simulink model "zad4_model"  (R2017a)
settings: Solver=VariableStepAuto  StartTime=0.0  StopTime=2  RelTol=1e-3
values from neighbouring files (symbols this model uses):
  a1 = Ap(1,1)    [zad4.m]
  a2 = Ap(2,1)    [zad4.m]
  a3 = Ap(3,1)    [zad4.m]
  b1 = Bp(1)    [zad4.m]
  b2 = Bp(2)    [zad4.m]
  b3 = Bp(3)    [zad4.m]
  K = acker(A2, B2, [z z z])    [zad3a.m]    (also in zad3b.m = acker(A2, B2, [z1 z2 z2]); zad3max.m; zad4.m = acker(Ap, Bp, [0.6 0.4 0.4]))
  l1 = L(1)    [zad4.m]
  l2 = L(2)    [zad4.m]
  Tp = 0.1    [zad3a.m]    (also in zad3b.m; zad3max.m; zad4.m)
settings Model: Creator=Rajtek  LastModifiedBy=Rajtek

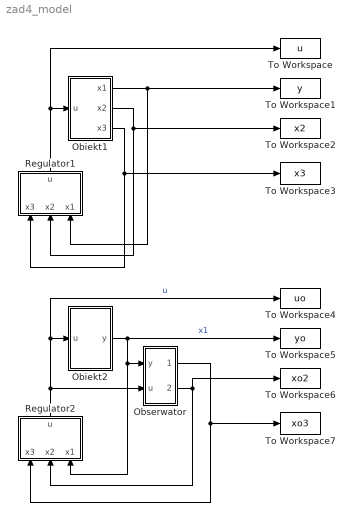
== system zad4_model ==
  Obiekt1 : Subsystem
  Obiekt2 : Subsystem
  Obserwator : Subsystem
  Regulator1 : Subsystem
  Regulator2 : Subsystem
  To Workspace : ToWorkspace  VariableName=u  SaveFormat=Timeseries  SampleTime=-1
  To Workspace1 : ToWorkspace  VariableName=y  SaveFormat=Timeseries  SampleTime=-1
  To Workspace2 : ToWorkspace  VariableName=x2  SaveFormat=Timeseries  SampleTime=-1
  To Workspace3 : ToWorkspace  VariableName=x3  SaveFormat=Timeseries  SampleTime=-1
  To Workspace4 : ToWorkspace  VariableName=uo  SaveFormat=Timeseries  SampleTime=-1
  To Workspace5 : ToWorkspace  VariableName=yo  SaveFormat=Timeseries  SampleTime=-1
  To Workspace6 : ToWorkspace  VariableName=xo2  SaveFormat=Timeseries  SampleTime=-1
  To Workspace7 : ToWorkspace  VariableName=xo3  SaveFormat=Timeseries  SampleTime=-1
  wires:
  Obiekt2/1(y) -> To Workspace5/1, Regulator2/3(x1), Obserwator/1(y)  "x1"
  Regulator2/1(u) -> To Workspace4/1, Obiekt2/1(u), Obserwator/2(u)  "u"
  Obserwator/1(xo3) -> Regulator2/1(x3), To Workspace7/1
  Obserwator/2(xo2) -> Regulator2/2(x2), To Workspace6/1
  Regulator1/1(u) -> To Workspace/1, Obiekt1/1(u)
  Obiekt1/1(x1) -> To Workspace1/1, Regulator1/3(x1)
  Obiekt1/2(x2) -> To Workspace2/1, Regulator1/2(x2)
  Obiekt1/3(x3) -> To Workspace3/1, Regulator1/1(x3)

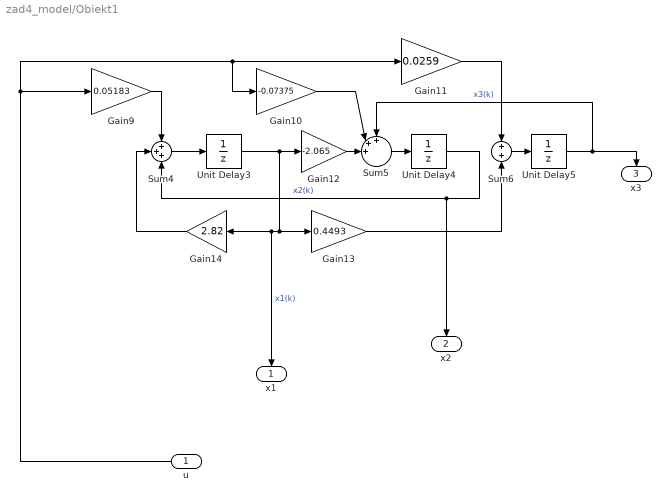
== system zad4_model/Obiekt1 ==
  u : Inport
  Gain10 : Gain  Gain=-0.07375
  Gain11 : Gain  Gain=0.0259
  Gain12 : Gain  Gain=-2.065
  Gain13 : Gain  Gain=0.4493
  Gain14 : Gain  Gain=2.82
  Gain9 : Gain  Gain=0.05183
  Sum4 : Sum  Inputs=+++
  Sum5 : Sum  Inputs=+++||
  Sum6 : Sum  Inputs=+|+
  Unit Delay3 : UnitDelay  InitialCondition=1  SampleTime=Tp
  Unit Delay4 : UnitDelay  InitialCondition=-2  SampleTime=Tp
  Unit Delay5 : UnitDelay  InitialCondition=2  SampleTime=Tp
  x1 : Outport
  x2 : Outport  Port=2
  x3 : Outport  Port=3
  wires:
  Sum6/1 -> Unit Delay5/1
  Sum5/1 -> Unit Delay4/1
  Gain11/1 -> Sum6/1
  Gain14/1 -> Sum4/2
  Gain13/1 -> Sum6/2
  Unit Delay5/1 -> x3/1, Sum5/1  "x3(k)"
  Sum4/1 -> Unit Delay3/1
  Gain9/1 -> Sum4/1
  Gain10/1 -> Sum5/2
  Gain12/1 -> Sum5/3
  Unit Delay4/1 -> x2/1, Sum4/3  "x2(k)"
  Unit Delay3/1 -> x1/1, Gain14/1, Gain13/1, Gain12/1  "x1(k)"
  u/1 -> Gain9/1, Gain11/1, Gain10/1

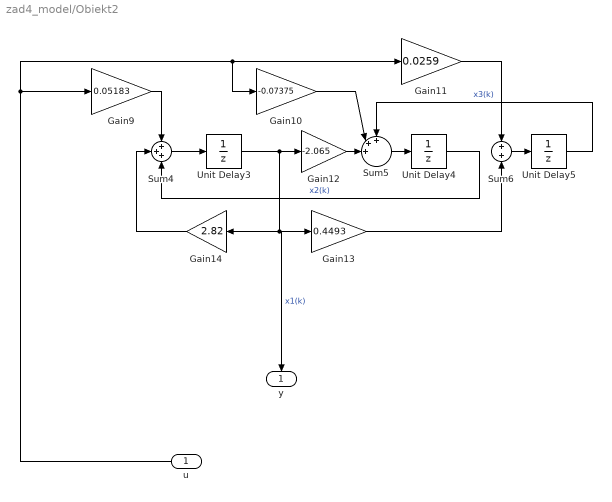
== system zad4_model/Obiekt2 ==
  u : Inport
  Gain10 : Gain  Gain=-0.07375
  Gain11 : Gain  Gain=0.0259
  Gain12 : Gain  Gain=-2.065
  Gain13 : Gain  Gain=0.4493
  Gain14 : Gain  Gain=2.82
  Gain9 : Gain  Gain=0.05183
  Sum4 : Sum  Inputs=+++
  Sum5 : Sum  Inputs=+++||
  Sum6 : Sum  Inputs=+|+
  Unit Delay3 : UnitDelay  InitialCondition=1  SampleTime=Tp
  Unit Delay4 : UnitDelay  InitialCondition=-2  SampleTime=Tp
  Unit Delay5 : UnitDelay  InitialCondition=2  SampleTime=Tp
  y : Outport
  wires:
  Sum6/1 -> Unit Delay5/1
  Sum5/1 -> Unit Delay4/1
  Gain11/1 -> Sum6/1
  Gain14/1 -> Sum4/2
  Gain13/1 -> Sum6/2
  Unit Delay5/1 -> Sum5/1  "x3(k)"
  Sum4/1 -> Unit Delay3/1
  Gain9/1 -> Sum4/1
  Gain10/1 -> Sum5/2
  Gain12/1 -> Sum5/3
  Unit Delay4/1 -> Sum4/3  "x2(k)"
  Unit Delay3/1 -> y/1, Gain13/1, Gain14/1, Gain12/1  "x1(k)"
  u/1 -> Gain9/1, Gain11/1, Gain10/1

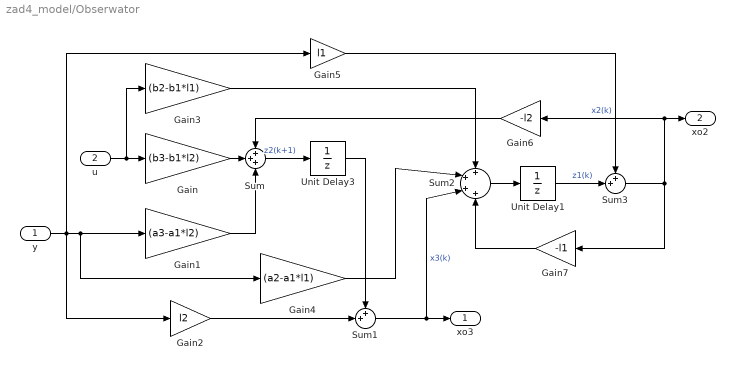
== system zad4_model/Obserwator ==
  y : Inport
  u : Inport  Port=2
  Gain : Gain  Gain=(b3-b1*l2)
  Gain1 : Gain  Gain=(a3-a1*l2)
  Gain2 : Gain  Gain=l2
  Gain3 : Gain  Gain=(b2-b1*l1)
  Gain4 : Gain  Gain=(a2-a1*l1)
  Gain5 : Gain  Gain=l1
  Gain6 : Gain  Gain=-l2
  Gain7 : Gain  Gain=-l1
  Sum : Sum  Inputs=+++
  Sum1 : Sum  Inputs=++|
  Sum2 : Sum  Inputs=++++
  Sum3 : Sum  Inputs=++|
  Unit Delay1 : UnitDelay  SampleTime=Tp
  Unit Delay3 : UnitDelay  SampleTime=Tp
  xo3 : Outport
  xo2 : Outport  Port=2
  wires:
  Gain1/1 -> Sum/3
  Unit Delay3/1 -> Sum1/1
  Gain6/1 -> Sum/1
  Sum3/1 -> Gain6/1, xo2/1, Gain7/1  "x2(k)"
  y/1 -> Gain5/1, Gain2/1, Gain4/1, Gain1/1
  u/1 -> Gain/1, Gain3/1
  Gain5/1 -> Sum3/1
  Gain7/1 -> Sum2/4
  Gain4/1 -> Sum2/2
  Sum/1 -> Unit Delay3/1  "z2(k+1)"
  Gain2/1 -> Sum1/2
  Gain/1 -> Sum/2
  Sum1/1 -> xo3/1, Sum2/3  "x3(k)"
  Unit Delay1/1 -> Sum3/2  "z1(k)"
  Gain3/1 -> Sum2/1
  Sum2/1 -> Unit Delay1/1

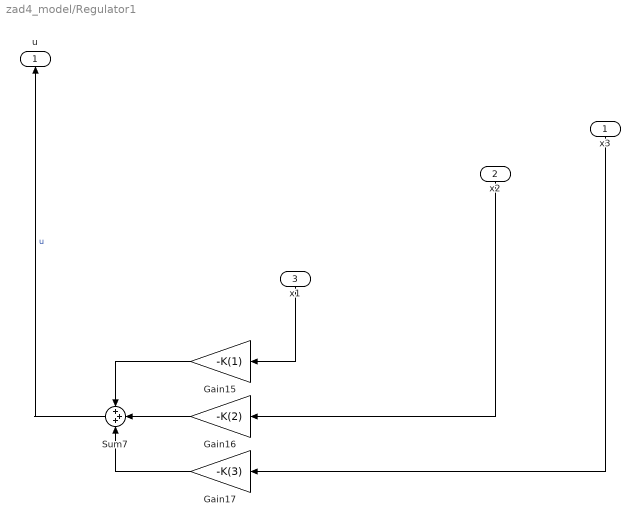
== system zad4_model/Regulator1 ==
  x3 : Inport
  x2 : Inport  Port=2
  x1 : Inport  Port=3
  Gain15 : Gain  Gain=-K(1)
  Gain16 : Gain  Gain=-K(2)
  Gain17 : Gain  Gain=-K(3)
  Sum7 : Sum  Inputs=+++
  u : Outport
  wires:
  Gain16/1 -> Sum7/2
  Gain17/1 -> Sum7/3
  Sum7/1 -> u/1  "u"
  Gain15/1 -> Sum7/1
  x3/1 -> Gain17/1
  x1/1 -> Gain15/1
  x2/1 -> Gain16/1

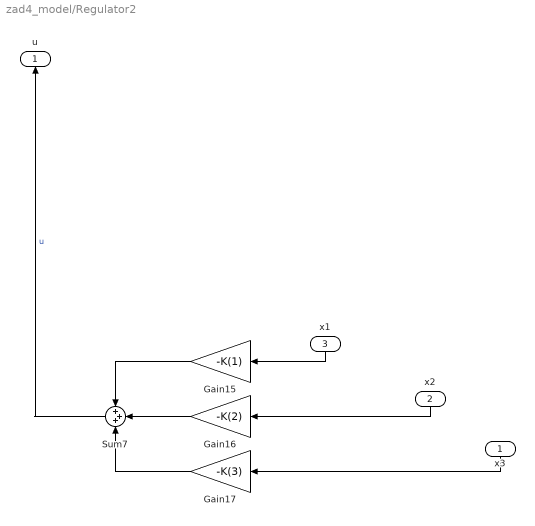
== system zad4_model/Regulator2 ==
  x3 : Inport
  x2 : Inport  Port=2
  x1 : Inport  Port=3
  Gain15 : Gain  Gain=-K(1)
  Gain16 : Gain  Gain=-K(2)
  Gain17 : Gain  Gain=-K(3)
  Sum7 : Sum  Inputs=+++
  u : Outport
  wires:
  Gain16/1 -> Sum7/2
  Gain17/1 -> Sum7/3
  Sum7/1 -> u/1  "u"
  Gain15/1 -> Sum7/1
  x3/1 -> Gain17/1
  x1/1 -> Gain15/1
  x2/1 -> Gain16/1
